simulink model "ODE_continuous"  (R2019b)
settings: Solver=FixedStepAuto  StartTime=0.0  StopTime=5  FixedStep=0.01  RelTol=1e-3
settings Model: Creator=Jieming  LastModifiedBy=sunji
settings DataIOCC: SaveFormat=Array  SaveState=on
settings SFSimCC: CustomCodeUndefinedFunction=UseInterfaceOnly

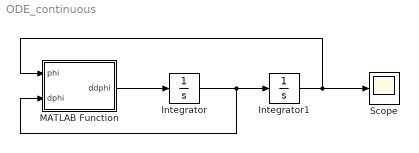
== system ODE_continuous ==
  Integrator : Integrator
  Integrator1 : Integrator
  MATLAB Function : MATLAB Function  TreatAsAtomicUnit=on
  Scope : Scope
  wires:
  MATLAB Function/1(ddphi) -> Integrator/1
  Integrator/1 -> MATLAB Function/2(dphi), Integrator1/1
  Integrator1/1 -> Scope/1, MATLAB Function/1(phi)

== matlab function ODE_continuous/MATLAB Function ==
  data: phi input; ddphi output; dphi input
function ddphi=   fcn(phi,dphi)
c1=4.2816*1e-7;
c2=1.568;
c3=5.7534;
h=80*1000/(4*pi)


ddphi= -c3*dphi+c2*cos(phi)+c1*h^2*sin(pi-2*phi);
